simulink model "fittsTask"  (R2012b)
settings: Solver=FixedStepDiscrete  StartTime=0.0  StopTime=10.0  FixedStep=0.001  RelTol=1e-3
undefined symbols (not defined in the file): autoplayMovementDuration, autoplayReactionTime, autoplayRotationDuration, autoplayRotationStart, clickPercentage, clickRefractoryPeriod, clickTargetColor, clickTargetHoverColor, cursorColorClick, cursorColorClosed, cursorColorOpen, cursorDiameter, delayOrder, displayObject, errorAssistAxis, errorAssistR, errorAssistTheta, expRandBinSize, expRandMax, expRandMin, expRandMu, failOnLiftoff, failurePenalty, falseClickFails, fingerPositionTolerance, gain, gloveBias, gloveLPDenominator, gloveLPNumerator, gloveNonlinearCorrection, gloveXCorrection, gloveYCorrection, gridEdges, gridTilesEachDim, holdDuration, holdTime, initialInput, inputType, lockFingerPosition, maxTaskTime, minTargetDistance, mouseLPDenominator, mouseLPNumerator, mouseOffset, movementDuration, movementOrder, numDisplayDims, numTargetDiameters, numTargets, numTrials, outputType, outputVelocityScaling, playSpokenCues, powerGain, powerGainUnityCrossing, preTrialLength, randomSeed, randomTaskBoundaries, randomTaskTargetDiameters, randomTaskTargetRotDiameters ... (+50)
settings Model: Creator=gilja  LastModifiedBy=NPTL
settings SolverCC: EnableConcurrentExecution=on  ConcurrentTasks=on
settings DataIOCC: SaveOutput=off  SignalLogging=off  SaveTime=off
settings OptimizationCC: InlineParams=on  InlineInvariantSignals=on  EnhancedBackFolding=on  EfficientFloat2IntCast=on  SimCompilerOptimization=On
settings DebuggingCC: UnderspecifiedInitializationDetection=Simplified
settings HardwareCC: ProdIntDivRoundTo=Zero  ProdEndianess=LittleEndian  ProdHWDeviceType=Generic->32-bit x86 compatible
settings ModelReferenceCC: ModelReferenceNumInstancesAllowed=Single  ModelReferenceMinAlgLoopOccurrences=on
settings RTWCC: SystemTargetFile=xpctarget.tlc  TemplateMakefile=xpc_default_tmf  Description=xPC Target  ProcessScript=xpctarget_make_rtw_hook  RTWCompilerOptimization=On
settings CodeAppCC: MaxIdLength=62
settings xpcTargetCC: TargetFcnLib=ansi_tfl_table_tmw.mat  CodeReplacementLibrary=XPC_BLAS  ParMdlRefBuildCompliant=on  ConcurrentExecutionCompliant=on  CombineSignalStateStructs=off  GRTInterface=on  xPCTaskExecutionProfile=on  xPCRL32EventNumber=5000  xPCisDownloadable=off  xPCLoadParamSetFile=off  xPCConcurrentTasks=off  xPCEnableSFAnimation=off

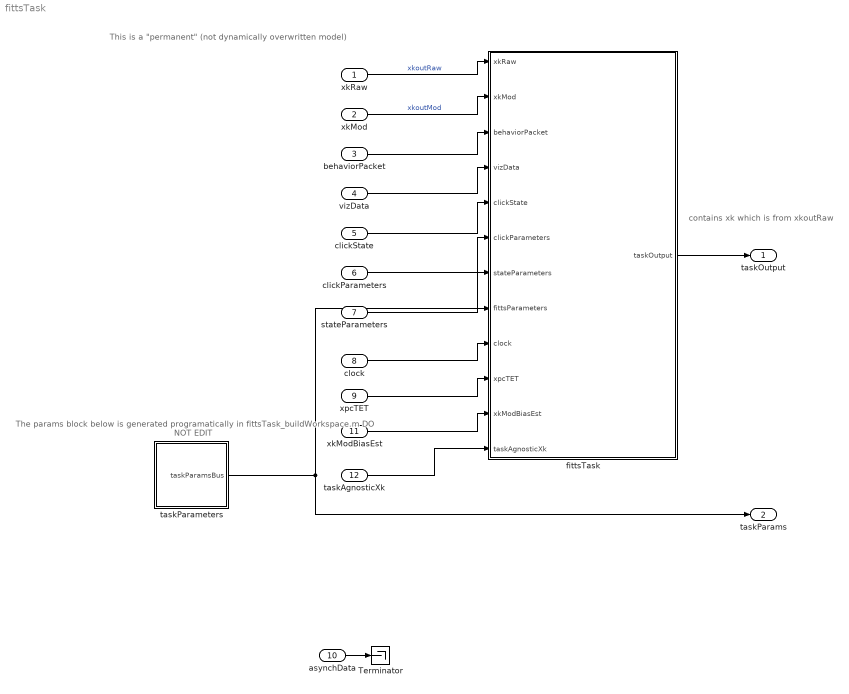
== system fittsTask ==
  note: contains xk which is
      | from xkoutRaw
  note: This is a "permanent" (not dynamically overwritten model)
  note: The params block below is generated programatically
      | in fittsTask_buildWorkspace.m
      | DO NOT EDIT
  xkRaw : Inport  OutDataTypeStr=double  PortDimensions=[double(xkConstants.NUM_STATE_DIMENSIONS),1]  SampleTime=[0.001,0]
  xkMod : Inport  Port=2  OutDataTypeStr=double  PortDimensions=[double(xkConstants.NUM_STATE_DIMENSIONS),1]  SampleTime=[0.001,0]
  behaviorPacket : Inport  Port=3  OutDataTypeStr=Bus: behaviorPacketBus
  vizData : Inport  Port=4  OutDataTypeStr=Bus: peripheralData  SampleTime=[0.001,0]
  clickState : Inport  Port=5  OutDataTypeStr=uint16  SampleTime=[0.001,0]
  clickParameters : Inport  Port=6  OutDataTypeStr=Bus: clickParametersBus
  stateParameters : Inport  Port=7  OutDataTypeStr=Bus: stateParams
  clock : Inport  Port=8  OutDataTypeStr=uint32  SampleTime=[0.001,0]
  xpcTET : Inport  Port=9  SampleTime=[0.001,0]
  asynchData : Inport  Port=10  OutDataTypeStr=Bus: peripheralData
  xkModBiasEst : Inport  Port=11  OutDataTypeStr=double  PortDimensions=[double(xkConstants.NUM_STATE_DIMENSIONS),1]  SampleTime=[0.001,0]
  taskAgnosticXk : Inport  Port=12  OutDataTypeStr=double  PortDimensions=[double(xkConstants.NUM_STATE_DIMENSIONS),1]  SampleTime=[0.001,0]
  Terminator : Terminator
  fittsTask : MATLAB Function  TreatAsAtomicUnit=on
  taskParameters : Subsystem
  taskOutput : Outport  OutDataTypeStr=Bus: taskOutput
  taskParams : Outport  Port=2  OutDataTypeStr=Bus: taskParamsBus  SampleTime=[0.001,0]
  wires:
  clickParameters/1 -> fittsTask/6(clickParameters)
  stateParameters/1 -> fittsTask/7(stateParameters)
  taskParameters/1(taskParamsBus) -> taskParams/1, fittsTask/8(fittsParameters)
  clock/1 -> fittsTask/9(clock)
  clickState/1 -> fittsTask/5(clickState)
  fittsTask/1(taskOutput) -> taskOutput/1
  xpcTET/1 -> fittsTask/10(xpcTET)
  vizData/1 -> fittsTask/4(vizData)
  behaviorPacket/1 -> fittsTask/3(behaviorPacket)
  asynchData/1 -> Terminator/1
  xkRaw/1 -> fittsTask/1(xkRaw)  "xkoutRaw"
  xkMod/1 -> fittsTask/2(xkMod)  "xkoutMod"
  xkModBiasEst/1 -> fittsTask/11(xkModBiasEst)
  taskAgnosticXk/1 -> fittsTask/12(taskAgnosticXk)

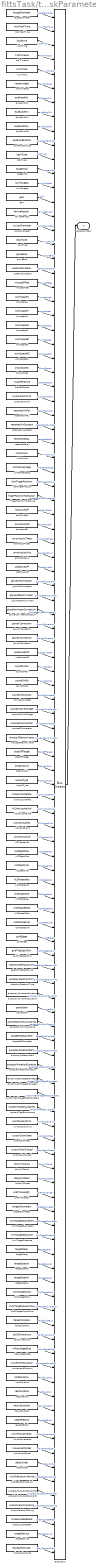
== system fittsTask/taskParameters ==
  BusOutput : BusCreator  Inputs=targetDiameter,maxTaskTime,holdTime,trialTimeout,numTrials,randomSeed,expRandMu,expRandMin,expRandMax,expRandBinSize,taskType,targetInds,numTargets,gain,failurePenalty,cursorDiameter,inputType,gloveBias,useRandomDelay,mouseOffset,workspaceX,workspaceY,workspaceZ,workspaceR,workspaceR2,showScores,trialsPerScore,cursorColorClick,recenterOnFail,recenterOnSuccess,recenterDelay,initialInput,clickPercentage,lockFingerPosition,fingerPositionTolerance,failOnLiftoff,errorAssistR,errorAssistTheta,errorAssistAxis,useGloveLPF,gloveLPNumerator,gloveLPDenominator,gloveNonlinearCorrection,gloveYCorrection,gloveXCorrection,useMouseLPF,soundOnFail,soundOnGo,soundOnSuccess,soundOnOverTarget,mouseLPNumerator,mouseLPDenominator,stopOffTarget,stopOnClick,outputType,xk2HorizontalPos,xk2HorizontalVel,xk2VerticalPos,xk2VerticalVel,xk2DepthPos,xk2DepthVel,xk2RotatePos,xk2RotateVel,xk2Rotate2Pos,xk2Rotate2Vel,gridEdges,gridTilesEachDim,selectionRefractoryMS,autoplayReactionTime,autoplayMovementDuration,powerGain,powerGainUnityCrossing,targetRotDiameter,autoplayRotationStart,autoplayRotationDuration,randomTaskTargetDiameters,randomTaskTargetRotDiameters,randomTaskBoundaries,numDisplayDims,cursorColorOpen,cursorColorClosed,showXYZaura,displayObject,preTrialLength,targetDiameters,numTargetDiameters,minTargetDistance,targetDelay,targetSpaceX,targetSpaceY,clickTargetColor,clickTargetHoverColor,falseClickFails,splitDimensions,xkRawSpeedCap,movementDuration,holdDuration,restDuration,returnDuration,repsPerBlock,whichMovements,movementOrder,delayOrder,clickRefractoryPeriod,xpcVelocityOutputPeriodMS,outputVelocityScaling,screenUpdateRate,targetDevice,playSpokenCues  OutDataTypeStr=Bus: taskParamsBus
  autoplayMovementDuration : Constant  Value=autoplayMovementDuration
  autoplayReactionTime : Constant  Value=autoplayReactionTime
  autoplayRotationDuration : Constant  Value=autoplayRotationDuration
  autoplayRotationStart : Constant  Value=autoplayRotationStart
  clickPercentage : Constant  Value=clickPercentage
  clickRefractoryPeriod : Constant  Value=clickRefractoryPeriod
  clickTargetColor : Constant  Value=clickTargetColor
  clickTargetHoverColor : Constant  Value=clickTargetHoverColor
  cursorColorClick : Constant  Value=cursorColorClick
  cursorColorClosed : Constant  Value=cursorColorClosed
  cursorColorOpen : Constant  Value=cursorColorOpen
  cursorDiameter : Constant  Value=cursorDiameter
  delayOrder : Constant  Value=delayOrder
  displayObject : Constant  Value=displayObject
  errorAssistAxis : Constant  Value=errorAssistAxis
  errorAssistR : Constant  Value=errorAssistR
  errorAssistTheta : Constant  Value=errorAssistTheta
  expRandBinSize : Constant  Value=expRandBinSize
  expRandMax : Constant  Value=expRandMax
  expRandMin : Constant  Value=expRandMin
  expRandMu : Constant  Value=expRandMu
  failOnLiftoff : Constant  Value=failOnLiftoff
  failurePenalty : Constant  Value=failurePenalty
  falseClickFails : Constant  Value=falseClickFails
  fingerPositionTolerance : Constant  Value=fingerPositionTolerance
  gain : Constant  Value=gain
  gloveBias : Constant  Value=gloveBias
  gloveLPDenominator : Constant  Value=gloveLPDenominator
  gloveLPNumerator : Constant  Value=gloveLPNumerator
  gloveNonlinearCorrection : Constant  Value=gloveNonlinearCorrection
  gloveXCorrection : Constant  Value=gloveXCorrection
  gloveYCorrection : Constant  Value=gloveYCorrection
  gridEdges : Constant  Value=gridEdges
  gridTilesEachDim : Constant  Value=gridTilesEachDim
  holdDuration : Constant  Value=holdDuration
  holdTime : Constant  Value=holdTime
  initialInput : Constant  Value=initialInput
  inputType : Constant  Value=inputType
  lockFingerPosition : Constant  Value=lockFingerPosition
  maxTaskTime : Constant  Value=maxTaskTime
  minTargetDistance : Constant  Value=minTargetDistance
  mouseLPDenominator : Constant  Value=mouseLPDenominator
  mouseLPNumerator : Constant  Value=mouseLPNumerator
  mouseOffset : Constant  Value=mouseOffset
  movementDuration : Constant  Value=movementDuration
  movementOrder : Constant  Value=movementOrder
  numDisplayDims : Constant  Value=numDisplayDims
  numTargetDiameters : Constant  Value=numTargetDiameters
  numTargets : Constant  Value=numTargets
  numTrials : Constant  Value=numTrials
  outputType : Constant  Value=outputType
  outputVelocityScaling : Constant  Value=outputVelocityScaling
  playSpokenCues : Constant  Value=playSpokenCues
  powerGain : Constant  Value=powerGain
  powerGainUnityCrossing : Constant  Value=powerGainUnityCrossing
  preTrialLength : Constant  Value=preTrialLength
  randomSeed : Constant  Value=randomSeed
  randomTaskBoundaries : Constant  Value=randomTaskBoundaries
  randomTaskTargetDiameters : Constant  Value=randomTaskTargetDiameters
  randomTaskTargetRotDiameters : Constant  Value=randomTaskTargetRotDiameters
  recenterDelay : Constant  Value=recenterDelay
  recenterOnFail : Constant  Value=recenterOnFail
  recenterOnSuccess : Constant  Value=recenterOnSuccess
  repsPerBlock : Constant  Value=repsPerBlock
  restDuration : Constant  Value=restDuration
  returnDuration : Constant  Value=returnDuration
  screenUpdateRate : Constant  Value=screenUpdateRate
  selectionRefractoryMS : Constant  Value=selectionRefractoryMS
  showScores : Constant  Value=showScores
  showXYZaura : Constant  Value=showXYZaura
  soundOnFail : Constant  Value=soundOnFail
  soundOnGo : Constant  Value=soundOnGo
  soundOnOverTarget : Constant  Value=soundOnOverTarget
  soundOnSuccess : Constant  Value=soundOnSuccess
  splitDimensions : Constant  Value=splitDimensions
  stopOffTarget : Constant  Value=stopOffTarget
  stopOnClick : Constant  Value=stopOnClick
  targetDelay : Constant  Value=targetDelay
  targetDevice : Constant  Value=targetDevice
  targetDiameter : Constant  Value=targetDiameter
  targetDiameters : Constant  Value=targetDiameters
  targetInds : Constant  Value=targetInds
  targetRotDiameter : Constant  Value=targetRotDiameter
  targetSpaceX : Constant  Value=targetSpaceX
  targetSpaceY : Constant  Value=targetSpaceY
  taskType : Constant  Value=taskType
  trialTimeout : Constant  Value=trialTimeout
  trialsPerScore : Constant  Value=trialsPerScore
  useGloveLPF : Constant  Value=useGloveLPF
  useMouseLPF : Constant  Value=useMouseLPF
  useRandomDelay : Constant  Value=useRandomDelay
  whichMovements : Constant  Value=whichMovements
  workspaceR : Constant  Value=workspaceR
  workspaceR2 : Constant  Value=workspaceR2
  workspaceX : Constant  Value=workspaceX
  workspaceY : Constant  Value=workspaceY
  workspaceZ : Constant  Value=workspaceZ
  xk2DepthPos : Constant  Value=xk2DepthPos
  xk2DepthVel : Constant  Value=xk2DepthVel
  xk2HorizontalPos : Constant  Value=xk2HorizontalPos
  xk2HorizontalVel : Constant  Value=xk2HorizontalVel
  xk2Rotate2Pos : Constant  Value=xk2Rotate2Pos
  xk2Rotate2Vel : Constant  Value=xk2Rotate2Vel
  xk2RotatePos : Constant  Value=xk2RotatePos
  xk2RotateVel : Constant  Value=xk2RotateVel
  xk2VerticalPos : Constant  Value=xk2VerticalPos
  xk2VerticalVel : Constant  Value=xk2VerticalVel
  xkRawSpeedCap : Constant  Value=xkRawSpeedCap
  xpcVelocityOutputPeriodMS : Constant  Value=xpcVelocityOutputPeriodMS
  taskParamsBus : Outport
  wires:
  targetDiameter/1 -> BusOutput/1  "targetDiameter"
  maxTaskTime/1 -> BusOutput/2  "maxTaskTime"
  holdTime/1 -> BusOutput/3  "holdTime"
  trialTimeout/1 -> BusOutput/4  "trialTimeout"
  numTrials/1 -> BusOutput/5  "numTrials"
  randomSeed/1 -> BusOutput/6  "randomSeed"
  expRandMu/1 -> BusOutput/7  "expRandMu"
  expRandMin/1 -> BusOutput/8  "expRandMin"
  expRandMax/1 -> BusOutput/9  "expRandMax"
  expRandBinSize/1 -> BusOutput/10  "expRandBinSize"
  taskType/1 -> BusOutput/11  "taskType"
  targetInds/1 -> BusOutput/12  "targetInds"
  numTargets/1 -> BusOutput/13  "numTargets"
  gain/1 -> BusOutput/14  "gain"
  failurePenalty/1 -> BusOutput/15  "failurePenalty"
  cursorDiameter/1 -> BusOutput/16  "cursorDiameter"
  inputType/1 -> BusOutput/17  "inputType"
  gloveBias/1 -> BusOutput/18  "gloveBias"
  useRandomDelay/1 -> BusOutput/19  "useRandomDelay"
  mouseOffset/1 -> BusOutput/20  "mouseOffset"
  workspaceX/1 -> BusOutput/21  "workspaceX"
  workspaceY/1 -> BusOutput/22  "workspaceY"
  workspaceZ/1 -> BusOutput/23  "workspaceZ"
  workspaceR/1 -> BusOutput/24  "workspaceR"
  workspaceR2/1 -> BusOutput/25  "workspaceR2"
  showScores/1 -> BusOutput/26  "showScores"
  trialsPerScore/1 -> BusOutput/27  "trialsPerScore"
  cursorColorClick/1 -> BusOutput/28  "cursorColorClick"
  recenterOnFail/1 -> BusOutput/29  "recenterOnFail"
  recenterOnSuccess/1 -> BusOutput/30  "recenterOnSuccess"
  recenterDelay/1 -> BusOutput/31  "recenterDelay"
  initialInput/1 -> BusOutput/32  "initialInput"
  clickPercentage/1 -> BusOutput/33  "clickPercentage"
  lockFingerPosition/1 -> BusOutput/34  "lockFingerPosition"
  fingerPositionTolerance/1 -> BusOutput/35  "fingerPositionTolerance"
  failOnLiftoff/1 -> BusOutput/36  "failOnLiftoff"
  errorAssistR/1 -> BusOutput/37  "errorAssistR"
  errorAssistTheta/1 -> BusOutput/38  "errorAssistTheta"
  errorAssistAxis/1 -> BusOutput/39  "errorAssistAxis"
  useGloveLPF/1 -> BusOutput/40  "useGloveLPF"
  gloveLPNumerator/1 -> BusOutput/41  "gloveLPNumerator"
  gloveLPDenominator/1 -> BusOutput/42  "gloveLPDenominator"
  gloveNonlinearCorrection/1 -> BusOutput/43  "gloveNonlinearCorrection"
  gloveYCorrection/1 -> BusOutput/44  "gloveYCorrection"
  gloveXCorrection/1 -> BusOutput/45  "gloveXCorrection"
  useMouseLPF/1 -> BusOutput/46  "useMouseLPF"
  soundOnFail/1 -> BusOutput/47  "soundOnFail"
  soundOnGo/1 -> BusOutput/48  "soundOnGo"
  soundOnSuccess/1 -> BusOutput/49  "soundOnSuccess"
  soundOnOverTarget/1 -> BusOutput/50  "soundOnOverTarget"
  mouseLPNumerator/1 -> BusOutput/51  "mouseLPNumerator"
  mouseLPDenominator/1 -> BusOutput/52  "mouseLPDenominator"
  stopOffTarget/1 -> BusOutput/53  "stopOffTarget"
  stopOnClick/1 -> BusOutput/54  "stopOnClick"
  outputType/1 -> BusOutput/55  "outputType"
  xk2HorizontalPos/1 -> BusOutput/56  "xk2HorizontalPos"
  xk2HorizontalVel/1 -> BusOutput/57  "xk2HorizontalVel"
  xk2VerticalPos/1 -> BusOutput/58  "xk2VerticalPos"
  xk2VerticalVel/1 -> BusOutput/59  "xk2VerticalVel"
  xk2DepthPos/1 -> BusOutput/60  "xk2DepthPos"
  xk2DepthVel/1 -> BusOutput/61  "xk2DepthVel"
  xk2RotatePos/1 -> BusOutput/62  "xk2RotatePos"
  xk2RotateVel/1 -> BusOutput/63  "xk2RotateVel"
  xk2Rotate2Pos/1 -> BusOutput/64  "xk2Rotate2Pos"
  xk2Rotate2Vel/1 -> BusOutput/65  "xk2Rotate2Vel"
  gridEdges/1 -> BusOutput/66  "gridEdges"
  gridTilesEachDim/1 -> BusOutput/67  "gridTilesEachDim"
  selectionRefractoryMS/1 -> BusOutput/68  "selectionRefractoryMS"
  autoplayReactionTime/1 -> BusOutput/69  "autoplayReactionTime"
  autoplayMovementDuration/1 -> BusOutput/70  "autoplayMovementDuration"
  powerGain/1 -> BusOutput/71  "powerGain"
  powerGainUnityCrossing/1 -> BusOutput/72  "powerGainUnityCrossing"
  targetRotDiameter/1 -> BusOutput/73  "targetRotDiameter"
  autoplayRotationStart/1 -> BusOutput/74  "autoplayRotationStart"
  autoplayRotationDuration/1 -> BusOutput/75  "autoplayRotationDuration"
  randomTaskTargetDiameters/1 -> BusOutput/76  "randomTaskTargetDiameters"
  randomTaskTargetRotDiameters/1 -> BusOutput/77  "randomTaskTargetRotDiameters"
  randomTaskBoundaries/1 -> BusOutput/78  "randomTaskBoundaries"
  numDisplayDims/1 -> BusOutput/79  "numDisplayDims"
  cursorColorOpen/1 -> BusOutput/80  "cursorColorOpen"
  cursorColorClosed/1 -> BusOutput/81  "cursorColorClosed"
  showXYZaura/1 -> BusOutput/82  "showXYZaura"
  displayObject/1 -> BusOutput/83  "displayObject"
  preTrialLength/1 -> BusOutput/84  "preTrialLength"
  targetDiameters/1 -> BusOutput/85  "targetDiameters"
  numTargetDiameters/1 -> BusOutput/86  "numTargetDiameters"
  minTargetDistance/1 -> BusOutput/87  "minTargetDistance"
  targetDelay/1 -> BusOutput/88  "targetDelay"
  targetSpaceX/1 -> BusOutput/89  "targetSpaceX"
  targetSpaceY/1 -> BusOutput/90  "targetSpaceY"
  clickTargetColor/1 -> BusOutput/91  "clickTargetColor"
  clickTargetHoverColor/1 -> BusOutput/92  "clickTargetHoverColor"
  falseClickFails/1 -> BusOutput/93  "falseClickFails"
  splitDimensions/1 -> BusOutput/94  "splitDimensions"
  xkRawSpeedCap/1 -> BusOutput/95  "xkRawSpeedCap"
  movementDuration/1 -> BusOutput/96  "movementDuration"
  holdDuration/1 -> BusOutput/97  "holdDuration"
  restDuration/1 -> BusOutput/98  "restDuration"
  returnDuration/1 -> BusOutput/99  "returnDuration"
  repsPerBlock/1 -> BusOutput/100  "repsPerBlock"
  whichMovements/1 -> BusOutput/101  "whichMovements"
  movementOrder/1 -> BusOutput/102  "movementOrder"
  delayOrder/1 -> BusOutput/103  "delayOrder"
  clickRefractoryPeriod/1 -> BusOutput/104  "clickRefractoryPeriod"
  xpcVelocityOutputPeriodMS/1 -> BusOutput/105  "xpcVelocityOutputPeriodMS"
  outputVelocityScaling/1 -> BusOutput/106  "outputVelocityScaling"
  screenUpdateRate/1 -> BusOutput/107  "screenUpdateRate"
  targetDevice/1 -> BusOutput/108  "targetDevice"
  playSpokenCues/1 -> BusOutput/109  "playSpokenCues"
  BusOutput/1 -> taskParamsBus/1

== matlab function fittsTask/fittsTask ==
  data: xkRaw input double size=[double(xkConstants.NUM_STATE_DIMENSIONS) 1]; xkMod input; behaviorPacket input Bus: behaviorPacketBus size=1; vizData input Bus: peripheralData; clickState input; clickParameters input; taskOutput output Bus: taskOutput; stateParameters input Bus: stateParams size=1; fittsParameters input Bus: taskParamsBus; clock input; xpcTET input; xkModBiasEst input; taskAgnosticXk input
function taskOutput  = fittsTask(xkRaw, xkMod, behaviorPacket, vizData, clickState, clickParameters, stateParameters, fittsParameters, clock, xpcTET, xkModBiasEst, taskAgnosticXk)
%#codegen

mouse = behaviorPacket.mouse(1:6);
glove = behaviorPacket.glove(1:5);
behaviorRequestClock = behaviorPacket.xpcRequestClock;
peripheralTimestamp = behaviorPacket.peripheralTimestamp(1:16);


%% CONSTANTS
TASK_NAME = 'fitts';
VERSION_ID = single(3.001); % Changed August 23 2016; BJ: updated to 3.001 with splitting of xk into xkRaw and xkMod.
NUM_DIMS = uint8(cursorConstants.NUM_DIMENSIONS); % dimensionality of the task. August 2016 raised this from 2 to 3
STATEVEC_SIZE = double( xkConstants.NUM_STATE_DIMENSIONS ); % SDS July 2016
INIT_LENGTH = uint16(2000); %ms
PRE_TRIAL_LENGTH = uint16(20); %ms
INIT_TIME = uint32(2000);


%% INITIALIZE CURSOR TASK OUTPUT
fileLoggerData.data = uint8(zeros(1,1400));
fileLoggerData.dataLen = uint16(0);
fileLoggerData.fileName = uint8(zeros(1,20));
fileLoggerData.send = false;

fileLoggerFormat.format = uint8(zeros(1,1400));
fileLoggerFormat.formatLen = uint16(0);
fileLoggerFormat.fileName = uint8(zeros(1,20));

fileLoggerFormatAndData.format = fileLoggerFormat;
fileLoggerFormatAndData.data = fileLoggerData;


%% TASK DETAILS PACKET
taskOutput.flushFiles = false;
taskOutput.sendFormat = false;
taskOutput.taskDetails = fileLoggerFormat;
taskOutput.discrete = fileLoggerFormatAndData;
taskOutput.continuous = fileLoggerFormatAndData;
taskOutput.screen = fileLoggerFormatAndData;
taskOutput.sound = fileLoggerFormatAndData;
taskOutput.asynch = fileLoggerFormatAndData;
taskOutput.ttl = double(0);
taskOutput.xk = xkRaw;
taskOutput.inputType = fittsParameters.initialInput;
taskOutput.currentTarget = single(zeros([double(xkConstants.NUM_TARGET_DIMENSIONS) 1]));
taskOutput.state = uint16(0);
taskOutput.paused = false;
taskOutput.allowStop = true;
taskOutput.resetHMM = true;

taskOutput.taskDetails = packFileLoggerTaskDetails(TASK_NAME, VERSION_ID, ...
    'STATE_INIT', uint16(FittsStates.STATE_INIT), ...
    'STATE_PRE_TRIAL', uint16(FittsStates.STATE_PRE_TRIAL),...
    'STATE_NEW_TARGET', uint16(FittsStates.STATE_NEW_TARGET),...
    'STATE_MOVE', uint16(FittsStates.STATE_MOVE),...
    'STATE_ACQUIRE', uint16(FittsStates.STATE_ACQUIRE),...
    'STATE_SUCCESS', uint16(FittsStates.STATE_SUCCESS),...
    'STATE_FAIL', uint16(FittsStates.STATE_FAIL),...
    'STATE_CENTER_TARGET', uint16(FittsStates.STATE_CENTER_TARGET),...
    'STATE_END', uint16(FittsStates.STATE_END),...
    'STATE_RECENTER_DELAY', uint16(FittsStates.STATE_RECENTER_DELAY),...
    'TASK_FITTS', uint16(fittsConstants.TASK_FITTS), ...
    'NUM_DIMENSIONS', uint8(DecoderConstants.NUM_KINEMATIC_DIMENSIONS), ...
    'INPUT_TYPE_MOUSE_ABSOLUTE', uint8(cursorConstants.INPUT_TYPE_MOUSE_ABSOLUTE), ...
    'INPUT_TYPE_DECODE_V', uint8(cursorConstants.INPUT_TYPE_DECODE_V),...
    'CLICK_TYPE_NONE', uint8(clickConstants.CLICK_TYPE_NONE),...
    'CLICK_TYPE_GLOVE', uint8(clickConstants.CLICK_TYPE_GLOVE),...
    'CLICK_TYPE_NEURAL', uint8(clickConstants.CLICK_TYPE_NEURAL)...
);

%% DEFINE PERSISTENTS
persistent state vizPacket;
persistent pauseTriggered;
persistent stateTimer;
persistent holdTimer;
persistent cursorColors;

persistent targetDiameters numTargetDiameters minTargetDistance;
persistent currentTargetDiameter nextTargetDiameter cursorDiameter holdTime trialTimeout failurePenalty;
persistent numTrials taskType gain inputType;

persistent currentTarget;
persistent nextTarget;

persistent targetSizeInd;
persistent trialNum;
persistent trialDelayLength;
persistent mouseOffset;

persistent workspaceX workspaceY;
persistent targetSpaceX targetSpaceY;

persistent recenterOnFail recenterOnSuccess recenterDelay;
persistent initialInput taskInput;

persistent distanceToTarget targetAngle numAvailableAngles;

persistent lastSoundTime;
persistent lastSoundState;

persistent clickTargetColor;
persistent clickTargetHoverColor;
persistent currentTargetType nextTargetType;
persistent lockedParameters;

persistent totalTaskTime;

%% INITIALIZE PERSISTENTS
if(isempty(state))
    state = uint16(FittsStates.STATE_INIT);
    currentTarget = int16(zeros([double(xkConstants.NUM_TARGET_DIMENSIONS) 1]));
    nextTarget = int16(zeros([double(xkConstants.NUM_TARGET_DIMENSIONS) 1]));
    
    vizPacket = initVizPacket;
    stateTimer = uint16(0);
    holdTimer = uint16(0);
    pauseTriggered = true;
    cursorColors = double(zeros([3 2]));
    
    
    %% buffer all the parameters off the bus
    lockedParameters = fittsParameters;
    
    targetDiameters = lockedParameters.targetDiameters;
    currentTargetDiameter = lockedParameters.targetDiameters(1);
    nextTargetDiameter = lockedParameters.targetDiameters(1);
    numTargetDiameters = lockedParameters.numTargetDiameters;
    minTargetDistance = lockedParameters.minTargetDistance;
    cursorDiameter = lockedParameters.cursorDiameter;
    holdTime = lockedParameters.holdTime;
    trialTimeout = lockedParameters.trialTimeout;
    failurePenalty = lockedParameters.failurePenalty;
    numTrials = lockedParameters.numTrials;
    taskType = lockedParameters.taskType;
    inputType = lockedParameters.initialInput;
    taskInput = lockedParameters.inputType;
    mouseOffset =  lockedParameters.mouseOffset;
    
    trialDelayLength = lockedParameters.targetDelay;
    gain = lockedParameters.gain;
    workspaceX = lockedParameters.workspaceX;
    workspaceY = lockedParameters.workspaceY;
    targetSpaceX = lockedParameters.targetSpaceX;
    targetSpaceY = lockedParameters.targetSpaceY;

    recenterOnFail = lockedParameters.recenterOnFail;
    recenterOnSuccess = lockedParameters.recenterOnSuccess;
    recenterDelay = lockedParameters.recenterDelay;

    initialInput = lockedParameters.initialInput;
    
    trialNum = uint16(0);
    targetSizeInd = uint16(0);
    distanceToTarget = nan;
    targetAngle = nan;
    numAvailableAngles = uint16(0);
    
    lastSoundTime = clock;
    lastSoundState = uint8(FittsStates.SOUND_STATE_IDLE);

    clickTargetColor = fittsParameters.clickTargetColor;
    clickTargetHoverColor = fittsParameters.clickTargetHoverColor;
    currentTargetType = uint16(cursorConstants.TARGET_TYPE_DWELL);
    nextTargetType = uint16(cursorConstants.TARGET_TYPE_DWELL);
    
    totalTaskTime = uint32(0);
end

%% which state elements do I look to for the cursor's position? SDS July 2016
xk2HorizontalPos = uint8( lockedParameters.xk2HorizontalPos );
xk2VerticalPos = uint8( lockedParameters.xk2VerticalPos );
xk2HorizontalVel = uint8( lockedParameters.xk2HorizontalVel );
xk2VerticalVel = uint8( lockedParameters.xk2VerticalVel );
xk2DepthPos = uint8( lockedParameters.xk2DepthPos );
xk2DepthVel = uint8( lockedParameters.xk2DepthVel );
xk2RotatePos = uint8( lockedParameters.xk2RotatePos );
xk2RotateVel = uint8( lockedParameters.xk2RotateVel );
% use a variable to store what indices of xkRaw & xkMod we care about so it's
% easier to extend this code to more dims.
canBePosInds = [xk2HorizontalPos,xk2VerticalPos,xk2DepthPos,xk2RotatePos];
effectorPosInds = canBePosInds(1:NUM_DIMS);
canBeVelInds = [xk2HorizontalVel,xk2VerticalVel,xk2DepthVel,xk2RotateVel];
effectorVelInds = canBeVelInds(1:NUM_DIMS);
% effectorPos = xk(effectorPosInds);

cursorPosition = xkMod(effectorPosInds); % updates cursorPosition in task based on xkMod (because potentially modified by EA and gain)

%%
if(clock < INIT_TIME)
    pauseTriggered = true;
end

% We usually shouldn't write discrete data
writeDiscreteData = false;
writeContinuousData = true;

if(vizData.receive && (vizData.dataLen > 0 ))
    vizPacket = parseVizPacket(vizData.data);
end

isNeural = (uint16(inputType) == uint16(cursorConstants.INPUT_TYPE_DECODE_V));
isClicked = (uint16(clickState) == uint16(DiscreteStates.CLICK_MAIN));

%% set the cursor color 
if isClicked
    cursorColors(1:end,1) = [255; 0; 0;];
else
    if isNeural
        cursorColors(1:end,1) = [255; 255; 255;];
    else
        cursorColors(1:end,1) = [255; 133; 0];
    end
end
targetColor = 'g';

if ~pauseTriggered
    totalTaskTime = totalTaskTime+1;
end


%% Map decoded neural state xk to task
% SDS August 2016 during move to highD
% BJ Nov 2016: changed xk to xkMod

%% STATE MACHINE
switch state
    case {FittsStates.STATE_INIT}
        %% set all the persistents that may have been changed by user input
        pauseTriggered = stateParameters.pause;

        targetDiameters = fittsParameters.targetDiameters;
        numTargetDiameters = fittsParameters.numTargetDiameters;
        minTargetDistance = fittsParameters.minTargetDistance;
        cursorDiameter = fittsParameters.cursorDiameter;
        holdTime = fittsParameters.holdTime;
        trialTimeout = fittsParameters.trialTimeout;
        failurePenalty = fittsParameters.failurePenalty;
        trialDelayLength = fittsParameters.targetDelay;
        gain = fittsParameters.gain;
        numTrials = fittsParameters.numTrials;
        taskType = fittsParameters.taskType;
        taskInput = fittsParameters.inputType;
        workspaceX = fittsParameters.workspaceX;
        workspaceY = fittsParameters.workspaceY;
        targetSpaceX = fittsParameters.targetSpaceX;
        targetSpaceY = fittsParameters.targetSpaceY;

        recenterOnFail = fittsParameters.recenterOnFail;
        recenterOnSuccess = fittsParameters.recenterOnSuccess;
        recenterDelay = fittsParameters.recenterDelay;
        
        initialInput = fittsParameters.initialInput;
        mouseOffset =  fittsParameters.mouseOffset;
        lockedParameters = fittsParameters;
                
        %% have the random number generator continuously going
        junkVal = rand(1,1);

        inputType = initialInput;
        if ~pauseTriggered
            inputType = taskInput;
            stateTimer = stateTimer + 1;
        else
            cursorPosition = double(zeros(NUM_DIMS,1));
        end
        if stateTimer >= INIT_LENGTH
            stateTimer = uint16(0);
            trialNum = uint16(0);
            currentTarget = int16(zeros([double(xkConstants.NUM_TARGET_DIMENSIONS) 1]));
            state = uint16(FittsStates.STATE_CENTER_TARGET);            
        end
        
    case {FittsStates.STATE_CENTER_TARGET}
        stateTimer = stateTimer + 1;
        if isCursorOnTarget(cursorPosition, double(cursorDiameter)/2, currentTarget, double(currentTargetDiameter)/2)
            state = uint16(FittsStates.STATE_SUCCESS);
            stateTimer = uint16(0);
            lastSoundTime = clock;
            lastSoundState = uint8(FittsStates.SOUND_STATE_SUCCESS);
        end
        
    case {FittsStates.STATE_NEW_TARGET}
        stateTimer = stateTimer + 1;
        if stateTimer >= trialDelayLength
            %% great, present the new target now
            stateTimer = uint16(0);
            writeDiscreteData = true;
            currentTarget = nextTarget;
            currentTargetDiameter = nextTargetDiameter;
            
            currentTargetType = nextTargetType;
            
            if currentTargetType == cursorConstants.TARGET_TYPE_CLICK;
                state = uint16(FittsStates.STATE_MOVE_CLICK);
            elseif currentTargetType == cursorConstants.TARGET_TYPE_DWELL;
                state = uint16(FittsStates.STATE_MOVE);
            end
            
        elseif ~isCursorOnTarget(cursorPosition, double(cursorDiameter)/2,  currentTarget, double(currentTargetDiameter)/2)
            %% fail if cursor moves from target early
            state = uint16(FittsStates.STATE_FAIL);
            stateTimer = uint16(0);
            lastSoundTime = clock;
            lastSoundState = uint8(FittsStates.SOUND_STATE_FAIL);
        end

    case {FittsStates.STATE_MOVE}
        stateTimer = stateTimer + 1;
        if isCursorOnTarget(cursorPosition, double(cursorDiameter)/2,  currentTarget, double(currentTargetDiameter)/2)
            state = uint16(FittsStates.STATE_ACQUIRE);
            holdTimer = uint16(0);
        elseif stateTimer >= trialTimeout
            stateTimer = uint16(0);
            state = uint16(FittsStates.STATE_FAIL);
            lastSoundTime = clock;
            lastSoundState = uint8(FittsStates.SOUND_STATE_FAIL);
        end
        
        case {FittsStates.STATE_MOVE_CLICK}
            stateTimer = stateTimer + 1;
            targetColor = char(clickTargetColor);
            networkOutput.discrete.send = false;
            if isCursorOnTarget(xkMod, double(cursorDiameter)/2,  currentTarget, double(currentTargetDiameter)/2)
                state = uint16(FittsStates.STATE_HOVER);
                holdTimer = uint16(0);
            elseif stateTimer >= trialTimeout
                stateTimer = uint16(0);
                state = uint16(FittsStates.STATE_FAIL);
                lastSoundTime = clock;
                lastSoundState = uint8(FittsStates.SOUND_STATE_FAIL);
            end
            
        case {FittsStates.STATE_HOVER}
            stateTimer = stateTimer + 1;
            targetColor = char(clickTargetHoverColor);
            networkOutput.discrete.send = false;
            if clickState == uint16(DiscreteStates.CLICK_MAIN)
                holdTimer = holdTimer + 1;
                if holdTimer >= clickParameters.clickHoldTime
                    state = uint16(FittsStates.STATE_SUCCESS);
                    stateTimer = uint16(0);
                    lastSoundTime = clock;
                    lastSoundState = uint8(FittsStates.SOUND_STATE_SUCCESS);
                end
            elseif ~isCursorOnTarget(xkMod, double(cursorDiameter)/2,  currentTarget, double(currentTargetDiameter)/2)
                state = uint16(FittsStates.STATE_MOVE_CLICK);
                holdTimer = uint16(0);
            elseif stateTimer >= trialTimeout
                stateTimer = uint16(0);
                state = uint16(FittsStates.STATE_FAIL);
                lastSoundTime = clock;
                lastSoundState = uint8(FittsStates.SOUND_STATE_FAIL);
            else
                holdTimer = uint16(0);                
            end
        
    case {FittsStates.STATE_ACQUIRE}
        stateTimer = stateTimer + 1;
        holdTimer = holdTimer + 1;
        targetColor = 'b';
        if ~isCursorOnTarget(cursorPosition, double(cursorDiameter)/2, currentTarget, double(currentTargetDiameter)/2)
            state = uint16(FittsStates.STATE_MOVE);
            holdTimer = uint16(0);
        elseif holdTimer >= holdTime
            stateTimer = uint16(0);
            state = uint16(FittsStates.STATE_SUCCESS);
            lastSoundTime = clock;
            lastSoundState = uint8(FittsStates.SOUND_STATE_SUCCESS);
        end
        
    case {FittsStates.STATE_SUCCESS}
        inputType = taskInput;
        trialNum = trialNum+1;
        
        stateTimer = uint16(0);

        if recenterOnSuccess
            state = uint16(FittsStates.STATE_RECENTER_DELAY);
        else
            state = uint16(FittsStates.STATE_PRE_TRIAL);
        end        
        
        
    case {FittsStates.STATE_FAIL}
        stateTimer = stateTimer+1;
        if isCursorOnTarget(cursorPosition, double(cursorDiameter)/2, currentTarget, double(currentTargetDiameter)/2)
            holdTimer = holdTimer +1;
        else
            holdTimer = uint16(0);
        end
        if holdTimer >= failurePenalty
            trialNum = trialNum + 1;
            stateTimer = uint16(0);
            
            if recenterOnFail
                state = uint16(FittsStates.STATE_RECENTER_DELAY);
            else
                state = uint16(FittsStates.STATE_PRE_TRIAL);
            end
            
        end
        
    case {FittsStates.STATE_RECENTER_DELAY}
        if stateTimer == 0
            %BJ: reset both xkMod and xkRaw
            xkMod(effectorPosInds,1) = currentTarget(1:NUM_DIMS);
            xkMod(effectorVelInds,1) = 0;
            xkRaw(effectorPosInds,1) = currentTarget(1:NUM_DIMS);
            xkRaw(effectorVelInds,1) = 0;
        end
        stateTimer = stateTimer+1;
        if stateTimer >= recenterDelay
            stateTimer = uint16(0);
            state = uint16(FittsStates.STATE_PRE_TRIAL);
        end            
        
        
    case {FittsStates.STATE_PRE_TRIAL}
        
        %% capture pauses
        if stateTimer == 0
            pauseTriggered = stateParameters.pause;
            % grab parameters again
            lockedParameters = fittsParameters;
        end
        if ~pauseTriggered
            stateTimer = stateTimer + 1;
        end
        %% don't do this on 0, because if we're paused, 0 will occur many many times
        if stateTimer == 1
            %% CHOOSE PROPERTIES FOR THE NEXT TARGET

            %% TARGET DIAMETERS:
            targetSizeInd = uint16(1+floor(rand(1,1)*double(numTargetDiameters)));
            nextTargetDiameter = targetDiameters(1,targetSizeInd);

            %% see which angles are valid 
            numAngleDivisions = 36;
            validAngles = zeros([1,numAngleDivisions],'uint16');
            totalDistances = zeros([1,numAngleDivisions], 'double');
            anglesInDegrees = double(0): double(floor(360/numAngleDivisions)): double(360-1);
            
            xDistance = double(0);
            yDistance = double(0);
            totalDistance = double(0);
            
            for in = 1:numAngleDivisions
                nn = double(anglesInDegrees(in));
                %% find the distance from the current target to the closest bound point
                %% dist to left bound:
                xProj = double(cosd(nn));
                if xProj == 0
                    xDistance = inf;
                else
                    if xProj <0
                        whichXBound = 1;
                    else
                        whichXBound = 2;
                    end
                    xDistance = abs(double(targetSpaceX(whichXBound)) -double(currentTarget(1))) / abs(xProj);
                end
                yProj = double(sind(nn));
                if yProj == 0
                    yDistance = inf;
                else
                    if yProj <0
                        whichYBound = 1;
                    else
                        whichYBound = 2;
                    end
                    yDistance = abs(double(targetSpaceY(whichYBound)) -double(currentTarget(2))) / abs(yProj);
                end
                if xDistance > yDistance
                    totalDistance = yDistance;
                else
                    totalDistance = xDistance;
                end
                if totalDistance < minTargetDistance + nextTargetDiameter
                    validAngles(in) = uint16(0);
                    totalDistances(in) = nan;
                else
                    validAngles(in) = uint16(1);
                    totalDistances(in) = totalDistance;
                end
            end

            %% now pick an angle from the available angles
            numAvailableAngles = uint16(sum(double(validAngles)));
            whichAngle = uint16(1+floor(rand(1,1)*double(numAvailableAngles)));
            anglesChecked = 0;
            for in = 1:numAngleDivisions
                if validAngles(in)
                    anglesChecked = anglesChecked+1;
                    if anglesChecked == double(whichAngle)
                        angleIndex = double(in);
                        break;
                    end
                end
            end
            distanceToNextTarget = double(minTargetDistance)+double(nextTargetDiameter)/2+rand(1,1)*double(totalDistances(angleIndex)-minTargetDistance-nextTargetDiameter);
            nextTarget(1) = int16(double(currentTarget(1)) + double(distanceToNextTarget) * double(cosd(anglesInDegrees(angleIndex))));
            nextTarget(2) = int16(double(currentTarget(2)) + double(distanceToNextTarget) * double(sind(anglesInDegrees(angleIndex))));
            distanceToTarget = distanceToNextTarget;
            targetAngle = anglesInDegrees(angleIndex);

            %% if next target is click or dwell
            clickRand = rand(1,1);
            if clickRand < lockedParameters.clickPercentage
                nextTargetType = uint16(cursorConstants.TARGET_TYPE_CLICK);
            else
                nextTargetType = uint16(cursorConstants.TARGET_TYPE_DWELL);
            end
        
        end
        if stateTimer >= PRE_TRIAL_LENGTH
            if trialNum > numTrials
                %% are we done?
                state = uint16(FittsStates.STATE_END);
            else
                state = uint16(FittsStates.STATE_NEW_TARGET);
            end
            stateTimer = uint16(0);
        end
        
    case {FittsStates.STATE_END}
        stateTimer = stateTimer + 1;
end

if lockedParameters.maxTaskTime && totalTaskTime > lockedParameters.maxTaskTime
    state = uint16(FittsStates.STATE_END);
end

taskOutput.xk = xkRaw;
taskOutput.currentTarget = single(currentTarget(:,1));
taskOutput.state = state;

taskAgnosticVel = single(taskAgnosticXk(effectorVelInds)');

%% PACK DATA FOR UDP OUTPUT
taskOutput.continuous = packFileLoggerFormatAndData('continuous', ...
    TASK_NAME, VERSION_ID, ...
    'clock', clock, ...
    'pause', pauseTriggered, ...
    'xpcRequestClock', behaviorPacket.xpcRequestClock, ...
    'state', state, ...
    'stateTimer', stateTimer, ...
    'inputType', inputType, ...
    'mouse', behaviorPacket.mouse, ...
    'glove', behaviorPacket.glove, ...
    'peripheralTimestamp', behaviorPacket.peripheralTimestamp,...
    'xpcScreenUpdateClock',vizPacket.xpcScreenUpdateClock,...
    'cursorPosition', single(cursorPosition), ...
    'currentTarget', int16(currentTarget(:,1)), ...
    'targetColor', targetColor,...
    'currentTargetDiameter', int16(currentTargetDiameter(:,1)), ...
    'xk', single(taskOutput.xk),...  %BJ: changed from xk to taskOutput.xk
    'stateTimer', stateTimer, ...
    'holdTimer', holdTimer, ...
    'xpcTET', single(xpcTET), ...
    'xkModBiasEst', single(xkModBiasEst), ...
    'taskAgnosticVel', taskAgnosticVel(1:NUM_DIMS) ...
    );




%% SEND DISCRETE DATA TO FILELOGGER
taskOutput.discrete = packFileLoggerFormatAndData('discrete', ...
    TASK_NAME, VERSION_ID, ...
    'clock', clock,...
    'state', state, ...
    'taskType', taskType, ...
    'currentTargetDiameter', currentTargetDiameter, ...
    'trialDelayLength', trialDelayLength, ...
    'gain', gain, ...
    'mouseOffset', mouseOffset, ...
    'currentTarget', currentTarget,...
    'trialNum', trialNum, ...
    'inputType', inputType, ...
    'workspaceX', workspaceX, ...
    'workspacey', workspaceY, ...
    'targetSpaceX', targetSpaceX, ...
    'targetSpaceY', targetSpaceY, ...
    'numTargetDiameters', numTargetDiameters, ...
    'targetDiameters', targetDiameters, ...
    'minTargetDistance', minTargetDistance, ...
    'targetAngle', targetAngle, ...
    'targetSizeInd', targetSizeInd, ...
    'distanceToTarget', distanceToTarget, ...
    'numAvailableAngles', numAvailableAngles, ...
    'recenterOnSuccess', recenterOnSuccess,...
    'recenterOnFail', recenterOnFail,...
    'errorAssistR',fittsParameters.errorAssistR,...    
    'errorAssistTheta',fittsParameters.errorAssistTheta,...    
    'clickPercentage',single(lockedParameters.clickPercentage),...
    'gloveThreshold', clickParameters.gloveThreshold, ...
    'gloveIndices', clickParameters.gloveIndices, ...
    'clickHoldTime', clickParameters.clickHoldTime, ...
    'clickSource', clickParameters.clickSource, ...
    'useGloveLPF', uint8(lockedParameters.useGloveLPF),...
    'hmmClickSpeedMax',single(clickParameters.hmmClickSpeedMax),...
    'recenterDelay', recenterDelay...
    );
%    'gloveLPNumerator', single(lockedParameters.gloveLPNumerator), ...
%    'gloveLPDenominator', single(lockedParameters.gloveLPNumerator), ...

    
%% SEND DATA OUT TO VIZ
taskOutput.screen = packFileLoggerFormatAndData('screen', ...
    TASK_NAME, VERSION_ID, ...
    'clock', clock,...
    'blockNumber', stateParameters.blockNumber,...
    'state',state,...
    'cursorPosition', cursorPosition,...
    'cursorColors', cursorColors,...
    'currentTarget', currentTarget,...
    'nextTarget', nextTarget,...
    'nextTargetDiameter', nextTargetDiameter,...
    'cursorDiameter', cursorDiameter,...
    'currentTargetDiameter', currentTargetDiameter,...
    'workspaceX', workspaceX,...
    'workspaceY',workspaceY,...
    'recenterDelay', recenterDelay...
    ); 

%% SEND DATA OUT TO SOUND
taskOutput.sound = packFileLoggerFormatAndData('screen', ...
    TASK_NAME, VERSION_ID, ...
    'clock', clock,...
    'vizState',state,...
    'lastSoundTime',lastSoundTime,...
    'lastSoundState',lastSoundState...
    ); 


%% SET SEND FLAGS FOR NETWORK OUTPUTS
if(clock < INIT_TIME)
    taskOutput.discrete.data.send = false;
    taskOutput.continuous.data.send = false;
    taskOutput.screen.data.send = false;
    taskOutput.sound.data.send = false;
    
    if(mod(clock, 10)==0)
        taskOutput.sendFormat = true;
    else
        taskOutput.sendFormat = false;
    end
    stateTimer = uint16(0);
else
    taskOutput.discrete.data.send = writeDiscreteData;
    taskOutput.continuous.data.send = writeContinuousData;
    taskOutput.screen.data.send = true;
    taskOutput.sound.data.send = true;
    taskOutput.sendFormat = false;
    taskOutput.inputType = inputType;
end
taskOutput.paused = pauseTriggered;
lastState = state;

end


function ccolor = updateCursorColor(inputType)
    switch inputType
        case fittsConstants.INPUT_TYPE_DECODE_V
                ccolor = [255; 255; 255;];
        otherwise
                ccolor = [255; 133; 0];
    end
end


function vizPacket = parseVizPacket(packetData)

    vizPacket.xpcScreenUpdateClock = typecast(packetData(28+[1:4]), 'uint32');

end

function vizPacket = initVizPacket()

    vizPacket.xpcScreenUpdateClock = uint32(0);

end




function icot = isCursorOnTarget(xkMod, cursorRadius, targetPosition, targetRadius)
    cursorPosition = xkMod(1:2);    %TODO: expand this check to be compatible with N-D
    if sqrt((double(cursorPosition(1)) - double(targetPosition(1))).^2 +...
            (double(cursorPosition(2)) - double(targetPosition(2))).^2) < double(cursorRadius+targetRadius)
        icot = true;
    else
        icot = false;
    end
    
end
